simulink model "chorus_try10sin"  (R2020b)
settings: Solver=VariableStepAuto  StartTime=0.0  StopTime=stop_time  RelTol=1e-3
InitFcn:
  | callback_init
StopFcn:
  | callback_stop
undefined symbols (not defined in the file): mp
libraries: dsphdlsigops x2, simulink x2, hdlsllib x2
settings Model: Creator=mvale_7a44q92  LastModifiedBy=mvale_7a44q92
settings DataIOCC: ReturnWorkspaceOutputs=off
settings OptimizationCC: BlockReduction=off  ConditionallyExecuteInputs=off  DefaultParameterBehavior=Inlined
settings DebuggingCC: AlgebraicLoopMsg=error
settings HardwareCC: ProdBitPerPointer=32  ProdBitPerSizeT=32  ProdBitPerPtrDiffT=32  ProdLargestAtomicFloat=None  ProdIntDivRoundTo=Undefined  ProdEndianess=Unspecified  ProdWordSize=32  ProdHWDeviceType=ASIC/FPGA->ASIC/FPGA  TargetBitPerPointer=64  TargetBitPerSizeT=64  TargetBitPerPtrDiffT=64  TargetLongLongMode=on  TargetIntDivRoundTo=Zero  TargetEndianess=LittleEndian  TargetWordSize=64  TargetHWDeviceType=Custom Processor->MATLAB Host Computer  ProdEqTarget=off

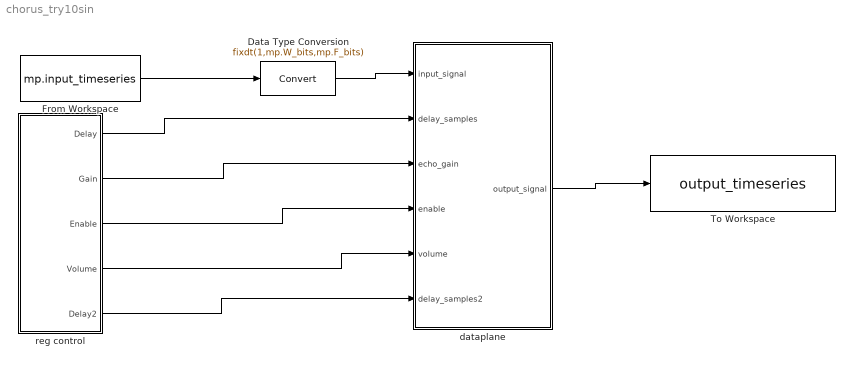
== system chorus_try10sin ==
  Data Type Conversion : DataTypeConversion  OutDataTypeStr=fixdt(1,mp.W_bits,mp.F_bits)
  From Workspace : FromWorkspace  VariableName=mp.input_timeseries  SampleTime=mp.Ts  OutputAfterFinalValue=Holding final value
  To Workspace : ToWorkspace  VariableName=output_timeseries  SaveFormat=Timeseries  SampleTime=-1
  dataplane : Subsystem
  reg control : Subsystem
  wires:
  From Workspace/1 -> Data Type Conversion/1
  dataplane/1(output_signal) -> To Workspace/1
  reg control/1(Delay) -> dataplane/2(delay_samples)
  reg control/2(Gain) -> dataplane/3(echo_gain)
  reg control/3(Enable) -> dataplane/4(enable)
  Data Type Conversion/1 -> dataplane/1(input_signal)
  reg control/4(Volume) -> dataplane/5(volume)
  reg control/5(Delay2) -> dataplane/6(delay_samples2)

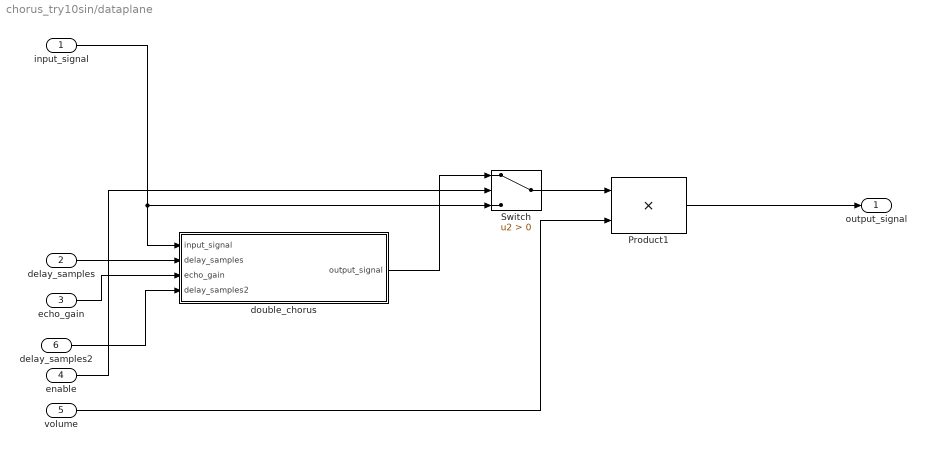
== system chorus_try10sin/dataplane ==
  input_signal : Inport
  delay_samples : Inport  Port=2
  echo_gain : Inport  Port=3
  enable : Inport  Port=4
  volume : Inport  Port=5
  delay_samples2 : Inport  Port=6
  Product1 : Product  OutDataTypeStr=Inherit: Same as first input
  Switch : Switch  Criteria=u2 > Threshold
  double_chorus : Subsystem
  output_signal : Outport
  wires:
  input_signal/1 -> Switch/3, double_chorus/1(input_signal)
  double_chorus/1(output_signal) -> Switch/1
  delay_samples/1 -> double_chorus/2(delay_samples)
  enable/1 -> Switch/2
  echo_gain/1 -> double_chorus/3(echo_gain)
  Switch/1 -> Product1/1
  Product1/1 -> output_signal/1
  volume/1 -> Product1/2
  delay_samples2/1 -> double_chorus/4(delay_samples2)

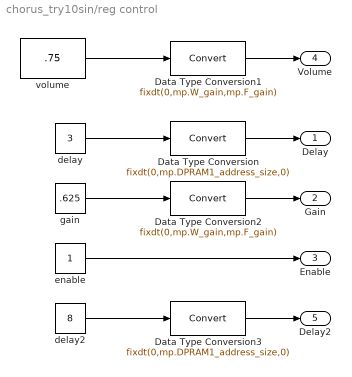
== system chorus_try10sin/reg control ==
  Data Type Conversion : DataTypeConversion  OutDataTypeStr=fixdt(0,mp.DPRAM1_address_size,0)
  Data Type Conversion1 : DataTypeConversion  OutMin=[0]  OutMax=[1]  OutDataTypeStr=fixdt(0,mp.W_gain,mp.F_gain)
  Data Type Conversion2 : DataTypeConversion  OutDataTypeStr=fixdt(0,mp.W_gain,mp.F_gain)
  Data Type Conversion3 : DataTypeConversion  OutDataTypeStr=fixdt(0,mp.DPRAM1_address_size,0)
  delay : Constant  Value=3  SampleTime=mp.Ts
  delay2 : Constant  Value=8  SampleTime=mp.Ts
  enable : Constant  OutDataTypeStr=boolean  SampleTime=mp.Ts
  gain : Constant  Value=.625  SampleTime=mp.Ts
  volume : Constant  Value=.75  SampleTime=mp.Ts
  Delay : Outport
  Gain : Outport  Port=2
  Enable : Outport  Port=3
  Volume : Outport  Port=4
  Delay2 : Outport  Port=5
  wires:
  delay/1 -> Data Type Conversion/1
  enable/1 -> Enable/1
  Data Type Conversion/1 -> Delay/1
  gain/1 -> Data Type Conversion2/1
  Data Type Conversion2/1 -> Gain/1
  volume/1 -> Data Type Conversion1/1
  Data Type Conversion1/1 -> Volume/1
  delay2/1 -> Data Type Conversion3/1
  Data Type Conversion3/1 -> Delay2/1

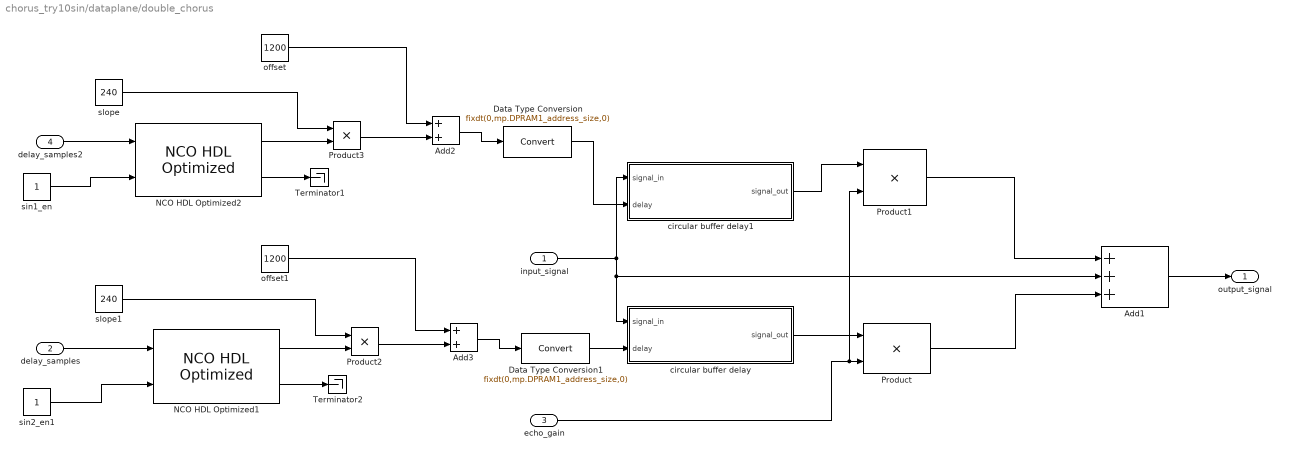
== system chorus_try10sin/dataplane/double_chorus ==
  input_signal : Inport
  delay_samples : Inport  Port=2
  echo_gain : Inport  Port=3
  delay_samples2 : Inport  Port=4
  Add1 : Sum  Inputs=+++  OutDataTypeStr=Inherit: Same as first input
  Add2 : Sum  OutDataTypeStr=fixdt(0,16,0)
  Add3 : Sum  OutDataTypeStr=fixdt(0,16,0)
  Data Type Conversion : DataTypeConversion  OutDataTypeStr=fixdt(0,mp.DPRAM1_address_size,0)
  Data Type Conversion1 : DataTypeConversion  OutDataTypeStr=fixdt(0,mp.DPRAM1_address_size,0)
  NCO HDL Optimized1 : dsphdlsigops/NCO HDL Optimized  PhaseIncrementSource=Input port  PhaseIncrement=100  PhaseOffsetSource=Property  PhaseOffset=0  DitherSource=Property  NumDitherBits=4  SamplesPerFrame=1  LUTCompress=off  ResetAction=off  Waveform=Sine  PhasePort=off  SimulateUsing=Code generation  AccumulatorWL=16  PhaseQuantization=on  NumQuantizerAccumulatorBits=12  OutputDataType=Binary point scaling  OutputWL=16  OutputFL=14
      settings: SourceProductName=DSP System Toolbox HDL Support
  NCO HDL Optimized2 : dsphdlsigops/NCO HDL Optimized  PhaseIncrementSource=Input port  PhaseIncrement=100  PhaseOffsetSource=Property  PhaseOffset=0  DitherSource=Property  NumDitherBits=4  SamplesPerFrame=1  LUTCompress=off  ResetAction=off  Waveform=Sine  PhasePort=off  SimulateUsing=Code generation  AccumulatorWL=16  PhaseQuantization=on  NumQuantizerAccumulatorBits=12  OutputDataType=Binary point scaling  OutputWL=16  OutputFL=14
      settings: SourceProductName=DSP System Toolbox HDL Support
  Product : Product  OutDataTypeStr=Inherit: Same as first input
  Product1 : Product  OutDataTypeStr=Inherit: Same as first input
  Product2 : Product  OutDataTypeStr=fixdt(0,16,0)
  Product3 : Product  OutDataTypeStr=fixdt(0,16,0)
  Terminator1 : Terminator
  Terminator2 : Terminator
  circular buffer delay : Subsystem
  circular buffer delay1 : Subsystem
  offset : Constant  Value=1200  OutDataTypeStr=fixdt(0,16,0)  SampleTime=mp.Ts
  offset1 : Constant  Value=1200  OutDataTypeStr=fixdt(0,16,0)  SampleTime=mp.Ts
  sin1_en : Constant  OutDataTypeStr=boolean  SampleTime=mp.Ts
  sin2_en1 : Constant  OutDataTypeStr=boolean  SampleTime=mp.Ts
  slope : Constant  Value=240  OutDataTypeStr=fixdt(0,16,0)  SampleTime=mp.Ts
  slope1 : Constant  Value=240  OutDataTypeStr=fixdt(0,16,0)  SampleTime=mp.Ts
  output_signal : Outport
  wires:
  Add1/1 -> output_signal/1
  input_signal/1 -> Add1/2, circular buffer delay/1(signal_in), circular buffer delay1/1(signal_in)
  echo_gain/1 -> Product1/2, Product/2
  circular buffer delay/1(signal_out) -> Product/1
  Product/1 -> Add1/3
  Product1/1 -> Add1/1
  circular buffer delay1/1(signal_out) -> Product1/1
  NCO HDL Optimized2/2 -> Terminator1/1
  Product3/1 -> Add2/2
  NCO HDL Optimized2/1 -> Product3/2
  Add2/1 -> Data Type Conversion/1
  delay_samples2/1 -> NCO HDL Optimized2/1
  Data Type Conversion/1 -> circular buffer delay1/2(delay)
  sin1_en/1 -> NCO HDL Optimized2/2
  NCO HDL Optimized1/2 -> Terminator2/1
  Product2/1 -> Add3/2
  Add3/1 -> Data Type Conversion1/1
  NCO HDL Optimized1/1 -> Product2/2
  Data Type Conversion1/1 -> circular buffer delay/2(delay)
  delay_samples/1 -> NCO HDL Optimized1/1
  sin2_en1/1 -> NCO HDL Optimized1/2
  slope/1 -> Product3/1
  offset/1 -> Add2/1
  slope1/1 -> Product2/1
  offset1/1 -> Add3/1

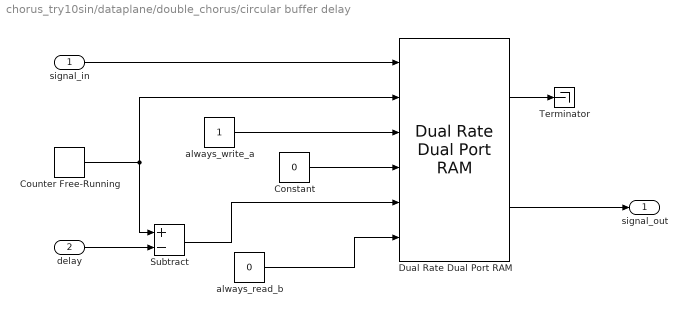
== system chorus_try10sin/dataplane/double_chorus/circular buffer delay ==
  signal_in : Inport
  delay : Inport  Port=2
  Constant : Constant  Value=0  OutDataTypeStr=fixdt(1,mp.W_bits,mp.F_bits)  SampleTime=mp.Ts
  Counter Free-Running : simulink/Sources/Counter Free-Running  NumBits=mp.DPRAM1_address_size  tsamp=mp.Ts
  Dual Rate Dual Port RAM : hdlsllib/HDL RAMs/Dual Rate Dual Port RAM  ram_size=mp.DPRAM1_address_size
      settings: SourceProductBaseCode=SL
  Subtract : Sum  Inputs=+-  OutDataTypeStr=Inherit: Same as first input
  Terminator : Terminator
  always_read_b : Constant  Value=0  OutDataTypeStr=boolean  SampleTime=mp.Ts
  always_write_a : Constant  OutDataTypeStr=boolean  SampleTime=mp.Ts
  signal_out : Outport
  wires:
  Subtract/1 -> Dual Rate Dual Port RAM/5
  signal_in/1 -> Dual Rate Dual Port RAM/1
  Constant/1 -> Dual Rate Dual Port RAM/4
  Counter Free-Running/1 -> Subtract/1, Dual Rate Dual Port RAM/2
  Dual Rate Dual Port RAM/2 -> signal_out/1
  always_write_a/1 -> Dual Rate Dual Port RAM/3
  always_read_b/1 -> Dual Rate Dual Port RAM/6
  delay/1 -> Subtract/2
  Dual Rate Dual Port RAM/1 -> Terminator/1

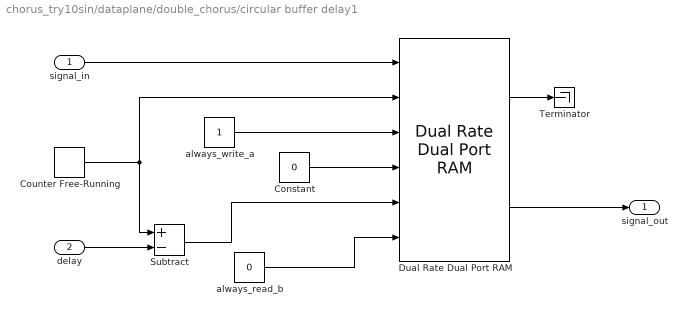
== system chorus_try10sin/dataplane/double_chorus/circular buffer delay1 ==
  signal_in : Inport
  delay : Inport  Port=2
  Constant : Constant  Value=0  OutDataTypeStr=fixdt(1,mp.W_bits,mp.F_bits)  SampleTime=mp.Ts
  Counter Free-Running : simulink/Sources/Counter Free-Running  NumBits=mp.DPRAM1_address_size  tsamp=mp.Ts
  Dual Rate Dual Port RAM : hdlsllib/HDL RAMs/Dual Rate Dual Port RAM  ram_size=mp.DPRAM1_address_size
      settings: SourceProductBaseCode=SL
  Subtract : Sum  Inputs=+-  OutDataTypeStr=Inherit: Same as first input
  Terminator : Terminator
  always_read_b : Constant  Value=0  OutDataTypeStr=boolean  SampleTime=mp.Ts
  always_write_a : Constant  OutDataTypeStr=boolean  SampleTime=mp.Ts
  signal_out : Outport
  wires:
  Subtract/1 -> Dual Rate Dual Port RAM/5
  signal_in/1 -> Dual Rate Dual Port RAM/1
  Constant/1 -> Dual Rate Dual Port RAM/4
  Counter Free-Running/1 -> Subtract/1, Dual Rate Dual Port RAM/2
  Dual Rate Dual Port RAM/2 -> signal_out/1
  always_write_a/1 -> Dual Rate Dual Port RAM/3
  always_read_b/1 -> Dual Rate Dual Port RAM/6
  delay/1 -> Subtract/2
  Dual Rate Dual Port RAM/1 -> Terminator/1
